simulink model "lab1sim"  (R2024a)
settings: Solver=VariableStepAuto  StartTime=0.0  StopTime=1000  RelTol=1e-3
libraries: simulink_extras x2, simulink x1
settings Model: Creator=Maryam  LastModifiedBy=Maryam

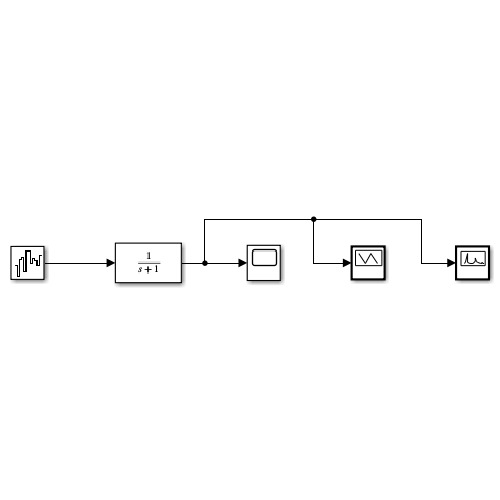
[thumbnail: Simulink's stored preview of the top-level diagram]
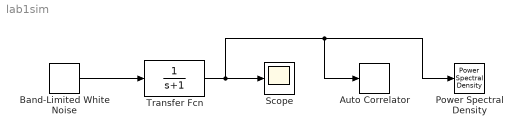
== system lab1sim ==
  Auto Correlator : simulink_extras/Additional Sinks/Auto Correlator  npts=100  HowOften=50  sampleT=0.1
  Band-Limited White Noise : simulink/Sources/Band-Limited White Noise  Cov=[0.1]  Ts=0.1  seed=[23341]
  Power Spectral Density : simulink_extras/Additional Sinks/Power Spectral Density  npts=128  fftpts=512  HowOften=64  sampleT=0.1
  Scope : Scope
  Transfer Fcn : TransferFcn  Denominator=[1 1]
  wires:
  Band-Limited White Noise/1 -> Transfer Fcn/1
  Transfer Fcn/1 -> Auto Correlator/1, Power Spectral Density/1, Scope/1
